simulink model "dual_hall_harmonic_baseline"  (R2024b)
settings: Solver=ode4  StartTime=0.0  StopTime=hall_t_stop_s  FixedStep=hall_ts_sim_s  RelTol=1e-3
model workspace (MAT data in the model file):
  hall_adc_bits = 16
  hall_amp_c_v = 0.85
  hall_amp_s_v = 1
  hall_amp_v = 1
  hall_angle_comp_orders = [1 2 3 4 5 6 7 8]
  hall_angle_fft_orders = [1 2 3 4 5 6 7 8 9 10 11 12]
  hall_f_mag_hz = 10
  hall_f_mech_hz = 1.66666666667
  hall_fig3_time_window_s = 0.5
  hall_harm_c_cos_v = [0.04 0.03 -0.018 0.013]
  hall_harm_c_sin_v = [-0.032 0.022 0.016 -0.012]
  hall_harm_orders = [2 3 5 6]
  hall_harm_s_cos_v = [0.018 0.028 -0.014 0.01]
  hall_harm_s_sin_v = [0.05 -0.035 0.024 0.016]
  hall_magnet_od_mm = 18
  hall_mech_speed_rpm = 100
  hall_offset_c_actual_v = 1.57
  hall_offset_err_c_v = -0.08
  hall_offset_err_s_v = 0.05
  hall_offset_s_actual_v = 1.7
  hall_offset_v = 1.65
  hall_omega_mech_rad_s = 10.471975512
  hall_phase_err_deg = 5
  hall_phase_err_rad = 0.0872664625997
  hall_pole_pairs = 6
  hall_signal_comp_orders = [2 3 5 6]
  hall_t_stop_s = 2
  hall_theta0_rad = 0
  hall_ts_sim_s = 0.0001
  hall_vref_v = 3.3
settings Model: Creator=26683  LastModifiedBy=26683

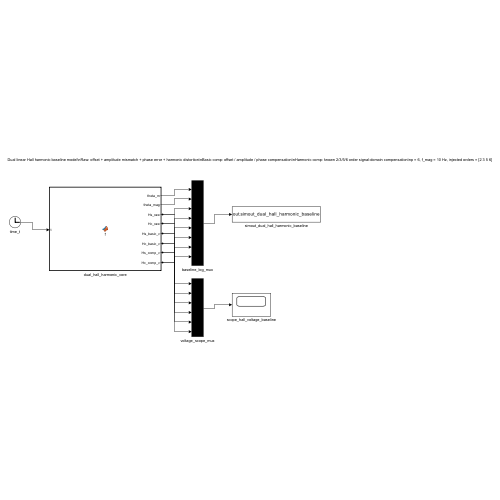
[thumbnail: Simulink's stored preview of the top-level diagram]
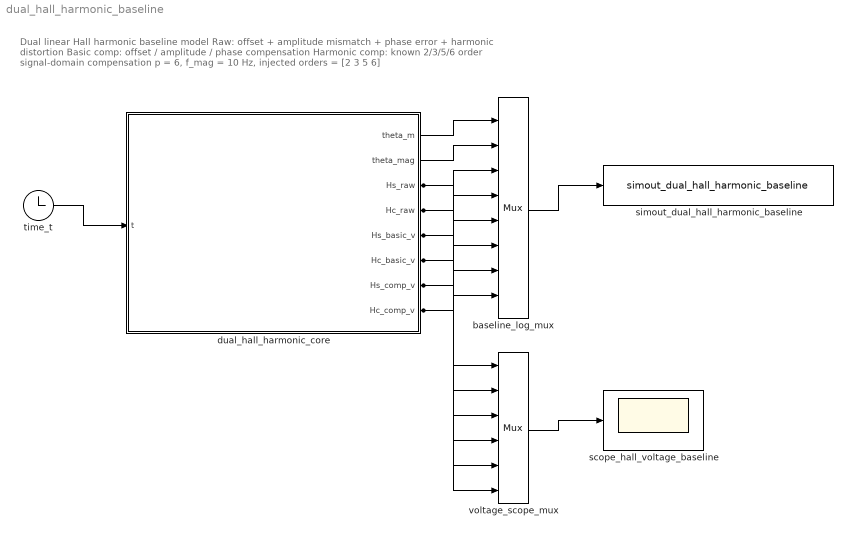
== system dual_hall_harmonic_baseline ==
  note: Dual linear Hall harmonic baseline model\nRaw: offset + amplitude mismatch + phase error + harmonic distortion\nBasic comp: offset / amplitude / phase compensation\nHarmonic comp: known 2/3/5/6 order signal-domain compensation\np = 6, f_mag = 10 Hz, injected orders = [2 3 5 6]
  baseline_log_mux : Mux  Inputs=8
  dual_hall_harmonic_core : MATLAB Function  TreatAsAtomicUnit=on
  scope_hall_voltage_baseline : Scope
  simout_dual_hall_harmonic_baseline : ToWorkspace  VariableName=simout_dual_hall_harmonic_baseline  SaveFormat=Structure With Time  SampleTime=-1
  time_t : Clock
  voltage_scope_mux : Mux  Inputs=6
  wires:
  time_t/1 -> dual_hall_harmonic_core/1(t)
  dual_hall_harmonic_core/1(theta_m) -> baseline_log_mux/1
  dual_hall_harmonic_core/2(theta_mag) -> baseline_log_mux/2
  dual_hall_harmonic_core/3(Hs_raw) -> baseline_log_mux/3, voltage_scope_mux/1
  dual_hall_harmonic_core/4(Hc_raw) -> baseline_log_mux/4, voltage_scope_mux/2
  dual_hall_harmonic_core/5(Hs_basic_v) -> baseline_log_mux/5, voltage_scope_mux/3
  dual_hall_harmonic_core/6(Hc_basic_v) -> baseline_log_mux/6, voltage_scope_mux/4
  dual_hall_harmonic_core/7(Hs_comp_v) -> baseline_log_mux/7, voltage_scope_mux/5
  dual_hall_harmonic_core/8(Hc_comp_v) -> baseline_log_mux/8, voltage_scope_mux/6
  baseline_log_mux/1 -> simout_dual_hall_harmonic_baseline/1
  voltage_scope_mux/1 -> scope_hall_voltage_baseline/1

== matlab function dual_hall_harmonic_baseline/dual_hall_harmonic_core ==
  data: t input; theta_m output; theta_mag output; Hs_raw output; Hc_raw output; Hs_basic_v output; Hc_basic_v output; Hs_comp_v output; Hc_comp_v output
function [theta_m, theta_mag, Hs_raw, Hc_raw, Hs_basic_v, Hc_basic_v, Hs_comp_v, Hc_comp_v] = f(t)
%#codegen
% 双线性霍尔谐波基准信号源。
% 该模块用已知注入参数演示 raw -> basic comp -> harmonic comp 的信号变化。
omega_m = 10.47197551196598;
pole_pairs = 6;
theta0 = 0;
offset_v = 1.65;
amp_nom_v = 1;
amp_s_v = 1;
amp_c_v = 0.85;
offset_s_v = 1.7;
offset_c_v = 1.57;
phase_err = 0.08726646259971647;
harm_orders = [2 3 5 6];
harm_s_sin = [0.05 -0.035 0.024 0.016];
harm_s_cos = [0.018 0.028 -0.014 0.01];
harm_c_sin = [-0.032 0.022 0.016 -0.012];
harm_c_cos = [0.04 0.03 -0.018 0.013];

theta_m = omega_m*t;
theta_mag = pole_pairs*theta_m + theta0;

Hs_harm = 0;
Hc_harm = 0;
for idx = 1:4
    n = harm_orders(idx);
    Hs_harm = Hs_harm + harm_s_sin(idx)*sin(n*theta_mag) + harm_s_cos(idx)*cos(n*theta_mag);
    Hc_harm = Hc_harm + harm_c_sin(idx)*sin(n*theta_mag) + harm_c_cos(idx)*cos(n*theta_mag);
end

Hs_raw = offset_s_v + amp_s_v*sin(theta_mag) + Hs_harm;
Hc_raw = offset_c_v + amp_c_v*cos(theta_mag + phase_err) + Hc_harm;

% 基础补偿：去除已知零偏和幅值不一致，并校正两路相位不正交。
xs_basic = (Hs_raw - offset_s_v)/amp_s_v;
xc_basic = (Hc_raw - offset_c_v)/amp_c_v;
xc_phasecorr = (xc_basic + xs_basic*sin(phase_err))/cos(phase_err);
Hs_basic_v = offset_v + amp_nom_v*xs_basic;
Hc_basic_v = offset_v + amp_nom_v*xc_phasecorr;

% 谐波补偿：扣除已知的信号域谐波残差，用于固定当前基准模型。
xs_harm_norm = Hs_harm/amp_s_v;
xc_harm_norm = Hc_harm/amp_c_v;
xc_harm_phasecorr = (xc_harm_norm + xs_harm_norm*sin(phase_err))/cos(phase_err);
xs_comp = xs_basic - xs_harm_norm;
xc_comp = xc_phasecorr - xc_harm_phasecorr;
Hs_comp_v = offset_v + amp_nom_v*xs_comp;
Hc_comp_v = offset_v + amp_nom_v*xc_comp;
